simulink model "MeanOE"  (R2018a)
settings: Solver=FixedStepAuto  StartTime=0.0  StopTime=stopTime  FixedStep=stepSize  RelTol=1e-3
values from neighbouring files (symbols this model uses):
  a_bar = mean(osc_a_J2)    [AA279D_PSET1.m]
  anom_bar = mean(osc_anom_J2)    [AA279D_PSET1.m]
  e_bar = mean(osc_e_J2)    [AA279D_PSET1.m]
  inc_bar = mean(osc_inc_J2)    [AA279D_PSET1.m]
  J2 = 1.081874*10^-3    (= 0.001081874)    [AA279D_PSET1.m]    (also in AA279D_PSET2.m; AA279D_PSET2_a_change.m)
  mu = 398600    [AA279D_PSET1.m]    (also in AA279D_PSET2.m; AA279D_PSET2_a_change.m; KeplerUniversalVsSTK.m = 398600.4418; TLE_Reader.m)
  RAAN_bar = mean(osc_RAAN_J2)    [AA279D_PSET1.m]
  Re = 6378137*10^-3    (= 6378.137)    [AA279D_PSET1.m]    (also in AA279D_PSET2.m; AA279D_PSET2_a_change.m)
  w_bar = mean(osc_w_J2)    [AA279D_PSET1.m]
settings Model: Creator=cwcovert  LastModifiedBy=Christopher Covert

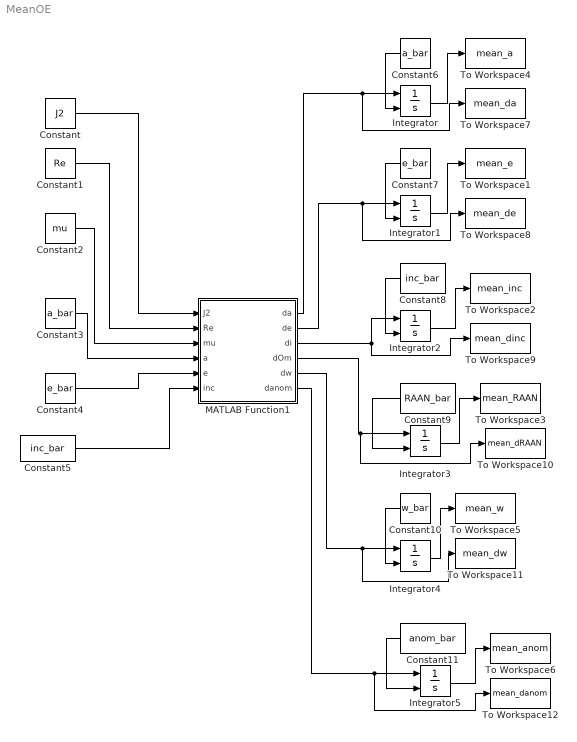
== system MeanOE ==
  Constant : Constant  Value=J2
  Constant1 : Constant  Value=Re
  Constant10 : Constant  Value=w_bar
  Constant11 : Constant  Value=anom_bar
  Constant2 : Constant  Value=mu
  Constant3 : Constant  Value=a_bar
  Constant4 : Constant  Value=e_bar
  Constant5 : Constant  Value=inc_bar
  Constant6 : Constant  Value=a_bar
  Constant7 : Constant  Value=e_bar
  Constant8 : Constant  Value=inc_bar
  Constant9 : Constant  Value=RAAN_bar
  Integrator{,1..5} (6 alike) : Integrator  InitialConditionSource=external
  MATLAB Function1 : MATLAB Function  TreatAsAtomicUnit=on
  To Workspace1 : ToWorkspace  VariableName=mean_e  SampleTime=-1
  To Workspace10 : ToWorkspace  VariableName=mean_dRAAN  SampleTime=-1
  To Workspace11 : ToWorkspace  VariableName=mean_dw  SampleTime=-1
  To Workspace12 : ToWorkspace  VariableName=mean_danom  SampleTime=-1
  To Workspace2 : ToWorkspace  VariableName=mean_inc  SampleTime=-1
  To Workspace3 : ToWorkspace  VariableName=mean_RAAN  SampleTime=-1
  To Workspace4 : ToWorkspace  VariableName=mean_a  SampleTime=-1
  To Workspace5 : ToWorkspace  VariableName=mean_w  SampleTime=-1
  To Workspace6 : ToWorkspace  VariableName=mean_anom  SampleTime=-1
  To Workspace7 : ToWorkspace  VariableName=mean_da  SampleTime=-1
  To Workspace8 : ToWorkspace  VariableName=mean_de  SampleTime=-1
  To Workspace9 : ToWorkspace  VariableName=mean_dinc  SampleTime=-1
  wires:
  Constant/1 -> MATLAB Function1/1(J2)
  Constant1/1 -> MATLAB Function1/2(Re)
  Constant2/1 -> MATLAB Function1/3(mu)
  Constant3/1 -> MATLAB Function1/4(a)
  Constant4/1 -> MATLAB Function1/5(e)
  Constant5/1 -> MATLAB Function1/6(inc)
  MATLAB Function1/1(da) -> To Workspace7/1, Integrator/1
  Integrator/1 -> To Workspace4/1
  Integrator1/1 -> To Workspace1/1
  MATLAB Function1/2(de) -> To Workspace8/1, Integrator1/1
  Integrator2/1 -> To Workspace2/1
  MATLAB Function1/3(di) -> To Workspace9/1, Integrator2/1
  Integrator3/1 -> To Workspace3/1
  MATLAB Function1/4(dOm) -> To Workspace10/1, Integrator3/1
  Integrator4/1 -> To Workspace5/1
  MATLAB Function1/5(dw) -> To Workspace11/1, Integrator4/1
  Integrator5/1 -> To Workspace6/1
  MATLAB Function1/6(danom) -> To Workspace12/1, Integrator5/1
  Constant6/1 -> Integrator/2
  Constant7/1 -> Integrator1/2
  Constant8/1 -> Integrator2/2
  Constant9/1 -> Integrator3/2
  Constant10/1 -> Integrator4/2
  Constant11/1 -> Integrator5/2

== matlab function MeanOE/MATLAB Function1 ==
  data: J2 input; da output; Re input; de output; mu input; di output; dOm output; dw output; danom output; a input; e input; inc input
function [da, de, di, dOm, dw, danom] = MeanOE(J2,Re,mu,a,e,inc)

p = a*(1-e^2);
n = sqrt(mu/a^3);
eta = sqrt(1-e^2);


da = 0;
de = 0;
di = 0;
dOm = -3/2*J2*(Re/p)^2*n*cosd(inc);
dw = 3/4*J2*(Re/p)^2*n*(5*cosd(inc)^2-1);
danom = 3/4*J2*(Re/p)^2*n*eta*(5*cosd(inc)^2-1);
